simulink model "main_SBus_pass_through"  (R2015a)
settings: Solver=ode3  StartTime=0.0  StopTime=time_end  FixedStep=time_step  RelTol=1e-3
libraries: dspnetwork x12, ec_arm_cortex_a_lib x1
settings Model: CovSFcnEnable=off  Creator=Magnus Blomberg  LastModifiedBy=Quad
settings DataIOCC: LimitDataPoints=off  MaxDataPoints=10000  SaveFormat=StructureWithTime  SignalLogging=off  SaveTime=off  ReturnWorkspaceOutputs=on
settings OptimizationCC: OptimizeModelRefInitCode=on  LifeSpan=Inf  MaxStackSize=64
settings DebuggingCC: SolverPrmCheckMsg=warning
settings HardwareCC: ProdLargestAtomicInteger=Long  ProdLargestAtomicFloat=Double  ProdEndianess=LittleEndian  ProdHWDeviceType=ARM Compatible->ARM Cortex
settings RTWCC: SystemTargetFile=ert.tlc  TLCOptions=-aInlineSetEventsForThisBaseRateFcn=TLC_FALSE -aSuppressMultiTaskScheduler=TLC_FALSE  TemplateMakefile=ert_default_tmf  Description=Embedded Coder  Toolchain=Linaro Toolchain v4.8
settings CodeAppCC: IgnoreCustomStorageClasses=off
settings ERTTargetCC: GenerateSampleERTMain=off  ParMdlRefBuildCompliant=on  CompOptLevelCompliant=on  ConcurrentExecutionCompliant=on  ERTFirstTimeCompliant=on  LogVarNameModifier=_rt  MatFileLogging=on  SupportContinuousTime=off  SupportVariableSizeSignals=off  ModelStepFunctionPrototypeControlCompliant=on  CPPClassGenCompliant=on  InlinedParameterPlacement=Hierarchical

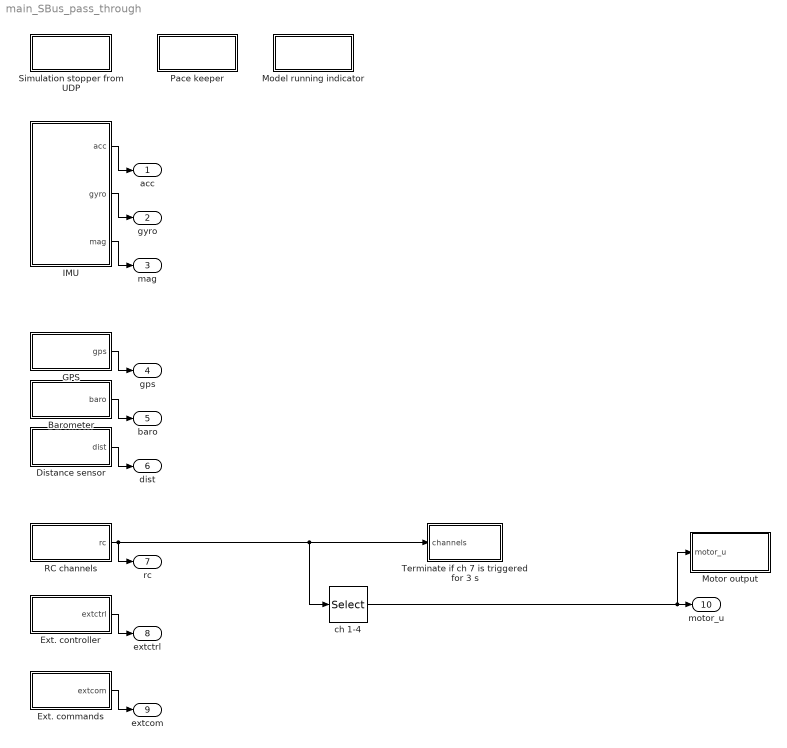
== system main_SBus_pass_through ==
  Barometer : Subsystem
  Distance sensor : Subsystem
  Ext. commands : Subsystem
  Ext. controller : Subsystem
  GPS : Subsystem
  IMU : Subsystem
  Model running indicator : Subsystem
  Motor output : Subsystem
  Pace keeper : Subsystem
  RC channels : Subsystem
  Simulation stopper from UDP : Subsystem
  Terminate if ch 7 is triggered for 3 s : Subsystem
  ch 1-4 : Selector  InputPortWidth=13  Indices=[1 2 3 4]
  acc : Outport
  gyro : Outport  Port=2
  mag : Outport  Port=3
  gps : Outport  Port=4
  baro : Outport  Port=5
  dist : Outport  Port=6
  rc : Outport  Port=7
  extctrl : Outport  Port=8
  extcom : Outport  Port=9
  motor_u : Outport  Port=10
  wires:
  IMU/1(acc) -> acc/1
  IMU/2(gyro) -> gyro/1
  IMU/3(mag) -> mag/1
  GPS/1(gps) -> gps/1
  Distance sensor/1(dist) -> dist/1
  RC channels/1(rc) -> rc/1, Terminate if ch 7 is triggered for 3 s/1(channels), ch 1-4/1
  Ext. controller/1(extctrl) -> extctrl/1
  Ext. commands/1(extcom) -> extcom/1
  Barometer/1(baro) -> baro/1
  ch 1-4/1 -> Motor output/1(motor_u), motor_u/1

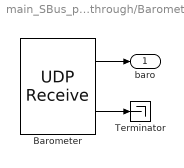
== system main_SBus_pass_through/Barometer ==
  Barometer : dspnetwork/UDP Receive  localURL='0.0.0.0'  localPort=22004  remoteURL='0.0.0.0'  remotePort=-1  recvBufferSize=8192  dims=3  signalDatatype=double  isVarSize=off  showBlockingTime=on  blockingTime=0  sampletime=0.02  blockPlatform=BeagleBone
  Terminator : Terminator
  baro : Outport
  wires:
  Barometer/2 -> Terminator/1
  Barometer/1 -> baro/1

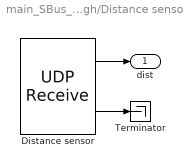
== system main_SBus_pass_through/Distance sensor ==
  Distance sensor : dspnetwork/UDP Receive  localURL='0.0.0.0'  localPort=22006  remoteURL='0.0.0.0'  remotePort=-1  recvBufferSize=8192  dims=3  signalDatatype=double  isVarSize=off  showBlockingTime=on  blockingTime=0  sampletime=0.02  blockPlatform=BeagleBone
  Terminator : Terminator
  dist : Outport
  wires:
  Distance sensor/2 -> Terminator/1
  Distance sensor/1 -> dist/1

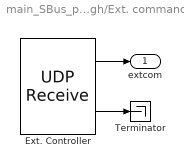
== system main_SBus_pass_through/Ext. commands ==
  Ext. Controller : dspnetwork/UDP Receive  localURL='0.0.0.0'  localPort=22201  remoteURL='0.0.0.0'  remotePort=-1  recvBufferSize=8192  dims=2  signalDatatype=double  isVarSize=off  showBlockingTime=on  blockingTime=0  sampletime=0.02  blockPlatform=BeagleBone
  Terminator : Terminator
  extcom : Outport
  wires:
  Ext. Controller/2 -> Terminator/1
  Ext. Controller/1 -> extcom/1

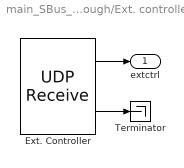
== system main_SBus_pass_through/Ext. controller ==
  Ext. Controller : dspnetwork/UDP Receive  localURL='0.0.0.0'  localPort=22102  remoteURL='0.0.0.0'  remotePort=-1  recvBufferSize=8192  dims=4  signalDatatype=double  isVarSize=off  showBlockingTime=on  blockingTime=0  sampletime=0.02  blockPlatform=BeagleBone
  Terminator : Terminator
  extctrl : Outport
  wires:
  Ext. Controller/2 -> Terminator/1
  Ext. Controller/1 -> extctrl/1

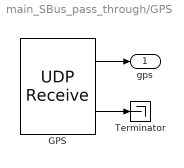
== system main_SBus_pass_through/GPS ==
  GPS : dspnetwork/UDP Receive  localURL='0.0.0.0'  localPort=22005  remoteURL='0.0.0.0'  remotePort=-1  recvBufferSize=8192  dims=3  signalDatatype=double  isVarSize=off  showBlockingTime=on  blockingTime=0  sampletime=0.02  blockPlatform=BeagleBone
  Terminator : Terminator
  gps : Outport
  wires:
  GPS/2 -> Terminator/1
  GPS/1 -> gps/1

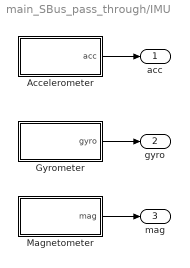
== system main_SBus_pass_through/IMU ==
  Accelerometer : Subsystem
  Gyrometer : Subsystem
  Magnetometer : Subsystem
  acc : Outport
  gyro : Outport  Port=2
  mag : Outport  Port=3
  wires:
  Magnetometer/1(mag) -> mag/1
  Gyrometer/1(gyro) -> gyro/1
  Accelerometer/1(acc) -> acc/1

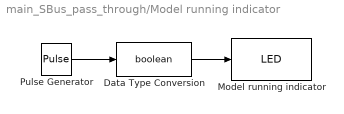
== system main_SBus_pass_through/Model running indicator ==
  Data Type Conversion : DataTypeConversion  OutDataTypeStr=boolean
  Model running indicator : ec_arm_cortex_a_lib/LED  board=BeagleBone Black  led=USR0  blockPlatform=BeagleBone
  Pulse Generator : DiscretePulseGenerator  PulseType=Time based  Period=.2  PulseWidth=50
  wires:
  Data Type Conversion/1 -> Model running indicator/1
  Pulse Generator/1 -> Data Type Conversion/1

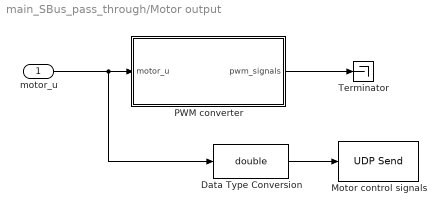
== system main_SBus_pass_through/Motor output ==
  motor_u : Inport
  Data Type Conversion : DataTypeConversion  OutDataTypeStr=double  LockScale=on
  Motor control signals : dspnetwork/UDP Send  remoteURL='127.0.0.1'  remotePort=25002  localURL='255.255.255.255'  localPortSource=Automatically determine  localPort=-1  sampletime=-1  blockPlatform=BeagleBone  separateLengthPort=0
  PWM converter : MATLAB Function  TreatAsAtomicUnit=on
  Terminator : Terminator
  wires:
  motor_u/1 -> Data Type Conversion/1, PWM converter/1(motor_u)
  PWM converter/1(pwm_signals) -> Terminator/1
  Data Type Conversion/1 -> Motor control signals/1

== system main_SBus_pass_through/Pace keeper ==
  Pac keeper : dspnetwork/UDP Send  remoteURL='127.0.0.1'  remotePort=25001  localURL='255.255.255.255'  localPortSource=Automatically determine  localPort=-1  sampletime=-1  blockPlatform=BeagleBone  separateLengthPort=0
  Pace constant : Constant  OutDataTypeStr=int8  SampleTime=Inf
  wires:
  Pace constant/1 -> Pac keeper/1

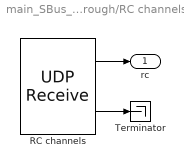
== system main_SBus_pass_through/RC channels ==
  RC channels : dspnetwork/UDP Receive  localURL='0.0.0.0'  localPort=22101  remoteURL='0.0.0.0'  remotePort=-1  recvBufferSize=200  dims=13  signalDatatype=double  isVarSize=off  showBlockingTime=on  blockingTime=1  sampletime=0.02  blockPlatform=BeagleBone
  Terminator : Terminator
  rc : Outport
  wires:
  RC channels/2 -> Terminator/1
  RC channels/1 -> rc/1

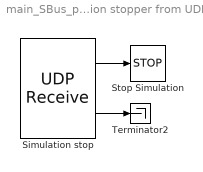
== system main_SBus_pass_through/Simulation stopper from UDP ==
  Simulation stop : dspnetwork/UDP Receive  localURL='0.0.0.0'  localPort=26001  remoteURL='0.0.0.0'  remotePort=-1  recvBufferSize=8192  dims=1  signalDatatype=boolean  isVarSize=off  showBlockingTime=on  blockingTime=0  sampletime=0.02  blockPlatform=BeagleBone
  Stop Simulation : Stop
  Terminator2 : Terminator
  wires:
  Simulation stop/1 -> Stop Simulation/1
  Simulation stop/2 -> Terminator2/1

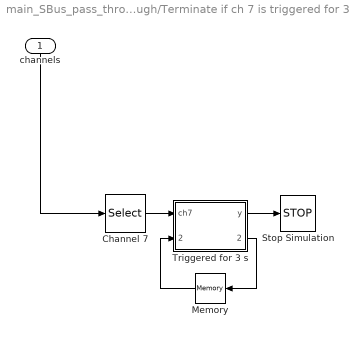
== system main_SBus_pass_through/Terminate if ch 7 is triggered for 3 s ==
  channels : Inport
  Channel 7 : Selector  InputPortWidth=13  Indices=[7]
  Memory : Memory
  Stop Simulation : Stop
  Triggered for 3 s : MATLAB Function  TreatAsAtomicUnit=on
  wires:
  Triggered for 3 s/1(y) -> Stop Simulation/1
  Channel 7/1 -> Triggered for 3 s/1(ch7)
  Memory/1 -> Triggered for 3 s/2(time_up_last)
  Triggered for 3 s/2(time_up) -> Memory/1
  channels/1 -> Channel 7/1

== system main_SBus_pass_through/IMU/Accelerometer ==
  Accelerometer : dspnetwork/UDP Receive  localURL='0.0.0.0'  localPort=22001  remoteURL='0.0.0.0'  remotePort=-1  recvBufferSize=8192  dims=3  signalDatatype=double  isVarSize=off  showBlockingTime=on  blockingTime=0  sampletime=0.02  blockPlatform=BeagleBone
  Terminator : Terminator
  acc : Outport
  wires:
  Accelerometer/2 -> Terminator/1
  Accelerometer/1 -> acc/1

== system main_SBus_pass_through/IMU/Gyrometer ==
  Gyrometer : dspnetwork/UDP Receive  localURL='0.0.0.0'  localPort=22002  remoteURL='0.0.0.0'  remotePort=-1  recvBufferSize=8192  dims=3  signalDatatype=double  isVarSize=off  showBlockingTime=on  blockingTime=0  sampletime=0.02  blockPlatform=BeagleBone
  Terminator : Terminator
  gyro : Outport
  wires:
  Gyrometer/2 -> Terminator/1
  Gyrometer/1 -> gyro/1

== system main_SBus_pass_through/IMU/Magnetometer ==
  Magnetometer : dspnetwork/UDP Receive  localURL='0.0.0.0'  localPort=22003  remoteURL='0.0.0.0'  remotePort=-1  recvBufferSize=8192  dims=3  signalDatatype=double  isVarSize=off  showBlockingTime=on  blockingTime=0  sampletime=0.02  blockPlatform=BeagleBone
  Terminator : Terminator
  mag : Outport
  wires:
  Magnetometer/2 -> Terminator/1
  Magnetometer/1 -> mag/1

== matlab function main_SBus_pass_through/Motor output/PWM converter ==
  data: motor_u input; pwm_signals output
function pwm_signals = fcn(motor_u)
%#codegen
pulse_min = 1100*1e-6;
pulse_max = 1930*1e-6;
pulse_f = 50;

pwm_signals = pulse_f * (pulse_min + motor_u .* (pulse_max - pulse_min));

== matlab function main_SBus_pass_through/Terminate if ch 7 is triggered for 3 s/Triggered for 3 s ==
  data: ch7 input; y output; time_up_last input; time_up output
function [y, time_up] = fcn(ch7, time_up_last)
y = 0;
time_step = 0.02;
if ch7 > 0.5
    time_up = time_up_last + time_step;
    if time_up > 3
        y = 1;
    end
else
    time_up = 0;
end
